simulink model "FIRST_ORDER"  (R2021a)
settings: Solver=VariableStepAuto  StartTime=0.0  StopTime=10.0  RelTol=1e-3
settings Model: Creator=Beshary  LastModifiedBy=Beshary

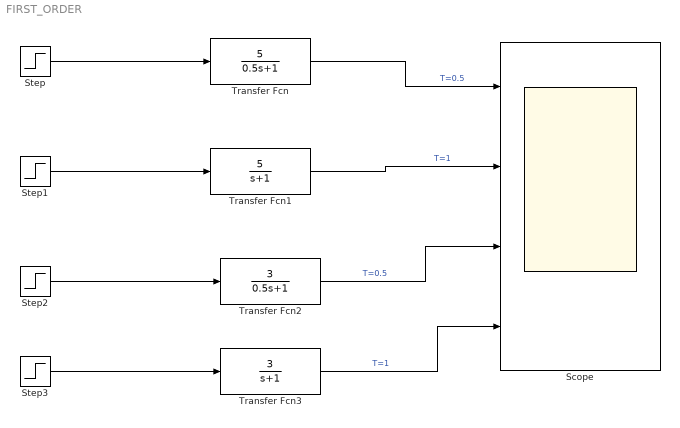
== system FIRST_ORDER ==
  Scope : Scope  NumInputPorts=4
  Step{,1..3} (4 alike) : Step  SampleTime=0
  Transfer Fcn : TransferFcn  Numerator=[5]  Denominator=[0.5 1]
  Transfer Fcn1 : TransferFcn  Numerator=[5]  Denominator=[1 1]
  Transfer Fcn2 : TransferFcn  Numerator=[3]  Denominator=[0.5 1]
  Transfer Fcn3 : TransferFcn  Numerator=[3]  Denominator=[1 1]
  wires:
  Step/1 -> Transfer Fcn/1
  Transfer Fcn/1 -> Scope/1  "T=0.5"
  Transfer Fcn1/1 -> Scope/2  "T=1"
  Step1/1 -> Transfer Fcn1/1
  Step2/1 -> Transfer Fcn2/1
  Transfer Fcn2/1 -> Scope/3  "T=0.5"
  Transfer Fcn3/1 -> Scope/4  "T=1"
  Step3/1 -> Transfer Fcn3/1
